simulink model "ley_de_control_minima_MGNLC"  (R2023b)
settings: Solver=VariableStepAuto  StartTime=0.0  StopTime=10.0  RelTol=1e-3
values from neighbouring files (symbols this model uses):
  L_q = 5.8e-3    (= 0.0058)    [diagrama_polos_y_ceros_LTI.m]    (also in main.m = 5.8; parametros.m; variacion_de_parametros.m)
  P_p = 3    [diagrama_polos_y_ceros_LTI.m]    (also in main.m; parametros.m; variacion_de_parametros.m)
settings Model: Creator=nicol  LastModifiedBy=nicol

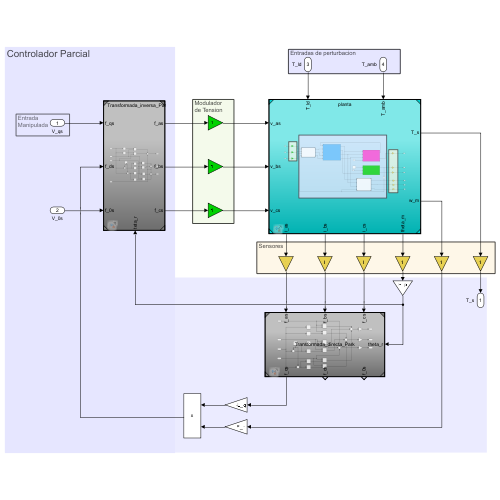
[thumbnail: Simulink's stored preview of the top-level diagram]
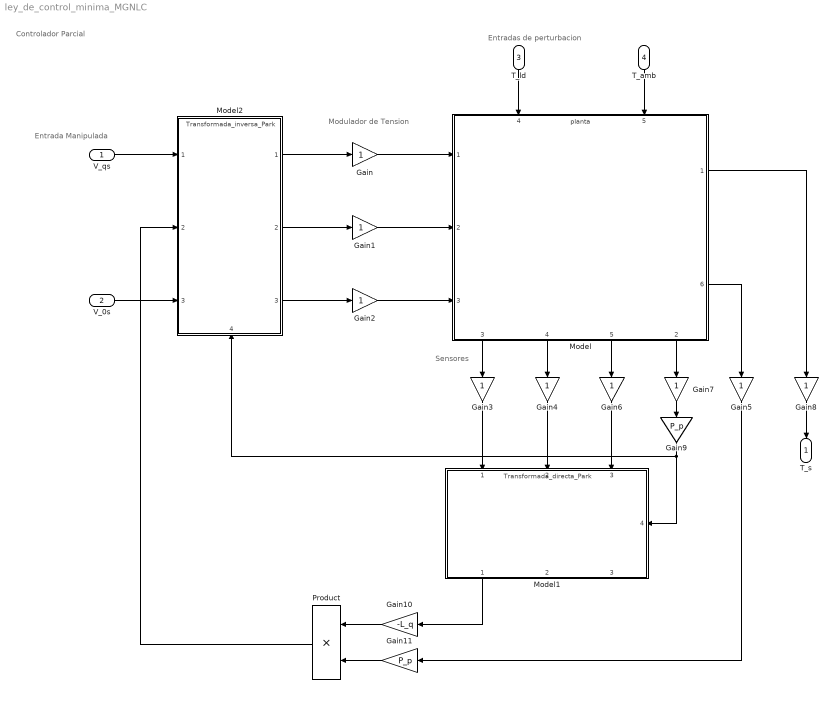
== system ley_de_control_minima_MGNLC ==
  note: Sensores
  note: Modulador
      | de Tension
  note: Entrada
      | Manipulada
  note: Entradas de perturbacion
  note: Controlador Parcial
  V_qs : Inport
  V_0s : Inport  Port=2
  T_ld : Inport  Port=3
  T_amb : Inport  Port=4
  Gain{,1..8} (9 alike) : Gain
  Gain10 : Gain  Gain=-L_q
  Gain11 : Gain  Gain=P_p
  Gain9 : Gain  Gain=P_p
  Model : ModelReference  ModelNameDialog=planta.slx  SimulationMode=Normal  ModelReferenceVersion=1.5
      settings: PortSchema="{\"entries\":[{\"content\":{\"sides\":[{\"content\":{\"connectorIds\":[\"In1\",\"In2\",\"In3\"]},\"type\":\"ConnectorPlacement.EquallySpacedRectSide\",\"uuid\":\"541f2dd0-63a5-498e-b6f4-429df3260999\"},{\"content\":{\"connectorIds\":[\"Out1\",\"Out6\"],\"side\":\"RIGHT\"},\"type\":\"ConnectorPlacement.EquallySpacedRectSide\",\"uuid\":\"3499a1c9-cb88-4d8d-9b35-501aa0f3df72\"},{\"content\":{\"connectorIds\":[\"In4\",\"In5\"],\"side\":\"TOP\"},\"type\":\"ConnectorPlacement.EquallySpacedRectSide\",\"uuid\":\"c32d79bf-ca05-414a-a73a-795c7b46d2b4\"},{\"content\":{\"connectorIds\":[\"Out3\",\"Out4\",\"Out5\",\"Out2\"],\"side\":\"BOTTOM\"},\"type\":\"ConnectorPlacement.EquallySpacedRectSide\",\"uuid\":\"087f7964-6389-41c1-86e8-9c28c159ac9c\"}]},\"type\":\"ConnectorPlacement.EquallySpacedConnector\",\"uuid\":\"654813cf-572e-4fc9-b0e4-bf7849c76800\"}],\"packageUris\":[\"http://schema.mathworks.com/mf0/Connector/R2020b\"],\"version\":\"1.0\"}"
  Model1 : ModelReference  ModelNameDialog=Transformada_directa_Park.slx  SimulationMode=Normal  ModelReferenceVersion=1.2
      settings: PortSchema="{\"entries\":[{\"content\":{\"sides\":[{\"content\":{\"connectorIds\":[\"In1\",\"In2\",\"In3\"]},\"type\":\"ConnectorPlacement.EquallySpacedRectSide\",\"uuid\":\"82c27493-c118-4c08-95af-31bb68eaa81e\"},{\"content\":{\"connectorIds\":[\"Out1\",\"Out2\",\"Out3\"],\"side\":\"RIGHT\"},\"type\":\"ConnectorPlacement.EquallySpacedRectSide\",\"uuid\":\"a10cc7bc-0b82-4cdd-8936-59a20eab3db5\"},{\"content\":{\"side\":\"TOP\"},\"type\":\"ConnectorPlacement.EquallySpacedRectSide\",\"uuid\":\"5ee0e5c4-eb4f-43d0-8f4c-35007b2184f0\"},{\"content\":{\"connectorIds\":[\"In4\"],\"side\":\"BOTTOM\"},\"type\":\"ConnectorPlacement.EquallySpacedRectSide\",\"uuid\":\"7c6f1f17-2c73-49cd-ba03-ecef4251f566\"}]},\"type\":\"ConnectorPlacement.EquallySpacedConnector\",\"uuid\":\"8bccd47c-0e45-48b8-8fad-d96c8b35cf51\"}],\"packageUris\":[\"http://schema.mathworks.com/mf0/Connector/R2020b\"],\"version\":\"1.0\"}"
  Model2 : ModelReference  ModelNameDialog=Transformada_inversa_Park.slx  SimulationMode=Normal  ModelReferenceVersion=1.3
      settings: PortSchema="{\"entries\":[{\"content\":{\"sides\":[{\"content\":{\"connectorIds\":[\"In1\",\"In2\",\"In3\"]},\"type\":\"ConnectorPlacement.EquallySpacedRectSide\",\"uuid\":\"82c27493-c118-4c08-95af-31bb68eaa81e\"},{\"content\":{\"connectorIds\":[\"Out1\",\"Out2\",\"Out3\"],\"side\":\"RIGHT\"},\"type\":\"ConnectorPlacement.EquallySpacedRectSide\",\"uuid\":\"a10cc7bc-0b82-4cdd-8936-59a20eab3db5\"},{\"content\":{\"side\":\"TOP\"},\"type\":\"ConnectorPlacement.EquallySpacedRectSide\",\"uuid\":\"5ee0e5c4-eb4f-43d0-8f4c-35007b2184f0\"},{\"content\":{\"connectorIds\":[\"In4\"],\"side\":\"BOTTOM\"},\"type\":\"ConnectorPlacement.EquallySpacedRectSide\",\"uuid\":\"7c065461-6f8e-43bc-bbfb-61ddb037de89\"}]},\"type\":\"ConnectorPlacement.EquallySpacedConnector\",\"uuid\":\"8bccd47c-0e45-48b8-8fad-d96c8b35cf51\"}],\"packageUris\":[\"http://schema.mathworks.com/mf0/Connector/R2020b\"],\"version\":\"1.0\"}"
  Product : Product
  T_s : Outport
  wires:
  Model2/1 -> Gain/1
  Model2/2 -> Gain1/1
  Model2/3 -> Gain2/1
  Gain2/1 -> Model/3
  Gain1/1 -> Model/2
  Gain/1 -> Model/1
  Gain4/1 -> Model1/2
  Model/4 -> Gain4/1
  Model/3 -> Gain3/1
  Gain3/1 -> Model1/1
  Model/5 -> Gain6/1
  Gain6/1 -> Model1/3
  Model/2 -> Gain7/1
  Model/6 -> Gain5/1
  Model/1 -> Gain8/1
  Gain9/1 -> Model1/4, Model2/4
  Gain7/1 -> Gain9/1
  Gain5/1 -> Gain11/1
  Model1/1 -> Gain10/1
  Gain11/1 -> Product/2
  Gain10/1 -> Product/1
  Product/1 -> Model2/2
  Gain8/1 -> T_s/1
  V_qs/1 -> Model2/1
  V_0s/1 -> Model2/3
  T_ld/1 -> Model/4
  T_amb/1 -> Model/5
